simulink library "Discrete_IO_Library_org"  (Simulink 10.0)
settings: Solver=ode45  StartTime=0.0  StopTime=10.0  RelTol=1e-3  EnableMultiTasking=on
libraries: $bdroot x3
settings Model: Creator=rruff  LastModifiedBy=bhisma

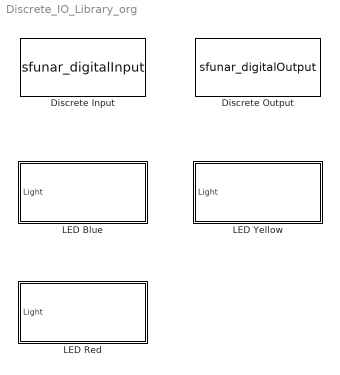
== system Discrete_IO_Library_org ==
  Discrete Input : S-Function  FunctionName=sfunar_digitalInput  Parameters=SParameter1, SampleTime  SFunctionDeploymentMode=off  EnableBusSupport=off  mask(ArduPilot Mega 2.0 Digital Input){SParameter1=2, SampleTime=0.1}
      mask prompts: SParameter1 "Pin Number:"; SampleTime "Sample time (-1 for inherited):"
      mask help:
      | Reads the digital value from the specified pin on the APM2 board.
      |
      | It outputs 1 for high and 0 for low.
      mask Help:
      | <p>This block calls the digitalRead() function from the Arduino language library.
      | <p>For more information see: <a href="http://arduino.cc/en/Reference/DigitalRead">Arduino - DigitalRead</a>
      mask Display:
      | text(.5,1,'ArduPilot Mega 2.0','horizontalAlignment','center','verticalAlignment','top');
      | plot([0 0.15 0.15 0.35 0.35 0.5],[0.3 0.3 0.7 0.7 0.3 0.3])
      | port_label('output',1,['Pin ', num2str(SParameter1)]);
  Discrete Output : S-Function  FunctionName=sfunar_digitalOutput  Parameters=uint8(SParameter1), SampleTime  SFunctionDeploymentMode=off  EnableBusSupport=off  mask(ArduPilot Mega 2.0 Digital Output){SParameter1=13, SampleTime=-1}
      mask prompts: SParameter1 "Pin Number:"; SampleTime "Sample time (-1 for inherited):"
      mask help:
      | Sends the digital value to the specified pin on the APM2 board.
      |
      | An input of 1 sets the pin high and 0 sets the pin low.
      mask Help:
      | <p>This block calls the digitalWrite() function from the Arduino language library.
      | <p>For more information see: <a href="http://arduino.cc/en/Reference/DigitalWrite">Arduino - DigitalWrite</a>
      mask Display:
      | text(.5,1,'ArduPilot Mega 2.0','horizontalAlignment','center','verticalAlignment','top');
      | plot([0.5 0.65 0.65 0.85 0.85 1],[0.3 0.3 0.7 0.7 0.3 0.3])
      | port_label('input',1,['Pin ', num2str(SParameter1)]);
  LED Blue : Subsystem  mask(ArduPilot Mega 2.0 Blue LED){}
      mask help: Controls the blue LED. Write 1 to turn on, 0 to turn off.
      mask Display:
      | text(.5,1,'ArduPilot Mega 2.0\nBlue LED','horizontalAlignment','center','verticalAlignment','top');
      | port_label('input', 1, 'On');
  LED Red : Subsystem  mask(ArduPilot Mega 2.0 Red LED){}
      mask help: Controls the red LED. Write 1 to turn on, 0 to turn off.
      mask Display:
      | text(.5,1,'ArduPilot Mega 2.0\nRed LED','horizontalAlignment','center','verticalAlignment','top');
      | port_label('input', 1, 'On');
  LED Yellow : Subsystem  mask(ArduPilot Mega 2.0 Yellow LED){}
      mask help: Controls the yellow LED. Write 1 to turn on, 0 to turn off.
      mask Display:
      | text(.5,1,'ArduPilot Mega 2.0\nYellow LED','horizontalAlignment','center','verticalAlignment','top');
      | port_label('input', 1, 'On');

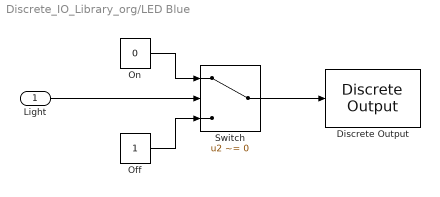
== system Discrete_IO_Library_org/LED Blue ==
  Light : Inport
  Discrete Output : $bdroot/Discrete Output  SParameter1=25  SampleTime=-1
  Off : Constant  OutDataTypeStr=uint8
  On : Constant  Value=0  OutDataTypeStr=uint8
  Switch : Switch  Criteria=u2 ~= 0
  wires:
  Light/1 -> Switch/2
  Switch/1 -> Discrete Output/1
  On/1 -> Switch/1
  Off/1 -> Switch/3

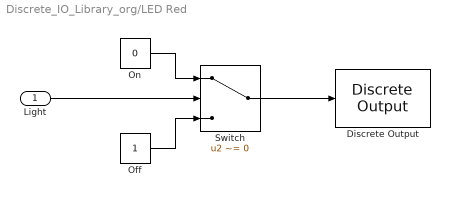
== system Discrete_IO_Library_org/LED Red ==
  Light : Inport
  Discrete Output : $bdroot/Discrete Output  SParameter1=27  SampleTime=-1
  Off : Constant  OutDataTypeStr=uint8
  On : Constant  Value=0  OutDataTypeStr=uint8
  Switch : Switch  Criteria=u2 ~= 0
  wires:
  Light/1 -> Switch/2
  Switch/1 -> Discrete Output/1
  On/1 -> Switch/1
  Off/1 -> Switch/3

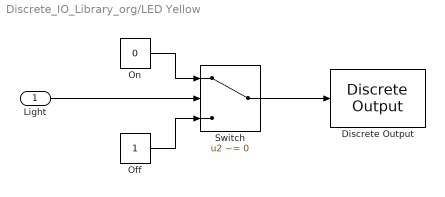
== system Discrete_IO_Library_org/LED Yellow ==
  Light : Inport
  Discrete Output : $bdroot/Discrete Output  SParameter1=26  SampleTime=-1
  Off : Constant  OutDataTypeStr=uint8
  On : Constant  Value=0  OutDataTypeStr=uint8
  Switch : Switch  Criteria=u2 ~= 0
  wires:
  Off/1 -> Switch/3
  On/1 -> Switch/1
  Switch/1 -> Discrete Output/1
  Light/1 -> Switch/2
